simulink model "parttwomodel"  (R2017b)
settings: Solver=VariableStepAuto  StartTime=0.0  StopTime=30000  RelTol=1e-3
undefined symbols (not defined in the file or in its folder): ain, aout, c, Kout, Qin
settings Model: Creator=justi  LastModifiedBy=justi

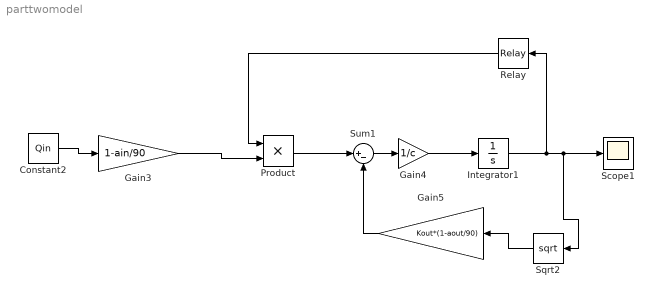
== system parttwomodel ==
  Constant2 : Constant  Value=Qin
  Gain3 : Gain  Gain=1-ain/90
  Gain4 : Gain  Gain=1/c
  Gain5 : Gain  Gain=Kout*(1-aout/90)
  Integrator1 : Integrator  InitialCondition=4
  Product : Product
  Relay : Relay
  Scope1 : Scope
  Sqrt2 : Sqrt  SaturateOnIntegerOverflow=on
  Sum1 : Sum  Inputs=|+-
  wires:
  Constant2/1 -> Gain3/1
  Gain3/1 -> Product/2
  Product/1 -> Sum1/1
  Sum1/1 -> Gain4/1
  Integrator1/1 -> Relay/1, Sqrt2/1, Scope1/1
  Gain4/1 -> Integrator1/1
  Gain5/1 -> Sum1/2
  Sqrt2/1 -> Gain5/1
  Relay/1 -> Product/1
